simulink model "freeEvolution"  (R2023b)
settings: Solver=VariableStepAuto  StartTime=0.0  StopTime=tf  RelTol=1e-6
values from neighbouring files (symbols this model uses):
  x0 = [deg2rad(10);0]    [ShipFinStabilizers.m]    (also in plotRoutine.m)
undefined symbols (not defined in the file or in its folder): A, B, C, D, F
settings Model: Creator=valen  LastModifiedBy=valen

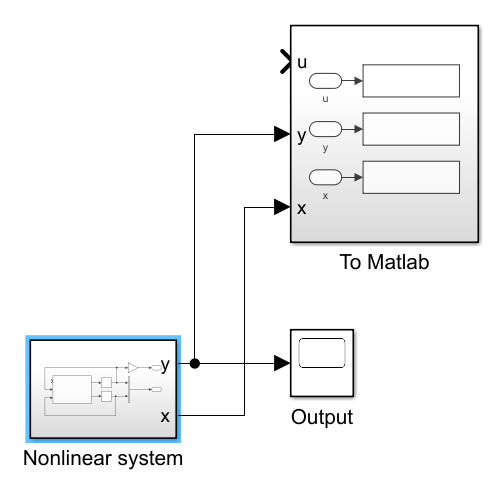
[thumbnail: Simulink's stored preview of the top-level diagram]
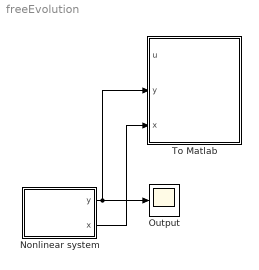
== system freeEvolution ==
  Nonlinear system : Subsystem
  Output : Scope
  To Matlab : Subsystem
  wires:
  Nonlinear system/2(x) -> To Matlab/3(x)
  Nonlinear system/1(y) -> To Matlab/2(y), Output/1

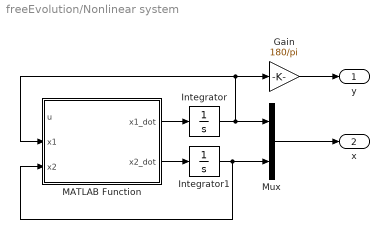
== system freeEvolution/Nonlinear system ==
  Gain : Gain  Gain=180/pi
  Integrator : Integrator  InitialCondition=x0(1)
  Integrator1 : Integrator  InitialCondition=x0(2)
  MATLAB Function : MATLAB Function  TreatAsAtomicUnit=on
  Mux : Mux  Inputs=2
  y : Outport
  x : Outport  Port=2
  wires:
  Integrator1/1 -> Mux/2, MATLAB Function/3(x2)
  Integrator/1 -> Mux/1, Gain/1, MATLAB Function/2(x1)
  MATLAB Function/2(x2_dot) -> Integrator1/1
  MATLAB Function/1(x1_dot) -> Integrator/1
  Mux/1 -> x/1
  Gain/1 -> y/1

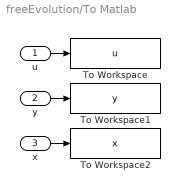
== system freeEvolution/To Matlab ==
  u : Inport  PortDimensions=1
  y : Inport  Port=2  PortDimensions=1
  x : Inport  Port=3  PortDimensions=[2,1]
  To Workspace : ToWorkspace  VariableName=u  SaveFormat=Structure With Time  SampleTime=-1
  To Workspace1 : ToWorkspace  VariableName=y  SaveFormat=Structure With Time  SampleTime=-1
  To Workspace2 : ToWorkspace  VariableName=x  SaveFormat=Structure With Time  SampleTime=-1
  wires:
  y/1 -> To Workspace1/1
  x/1 -> To Workspace2/1
  u/1 -> To Workspace/1

== matlab function freeEvolution/Nonlinear system/MATLAB Function ==
  data: u input; x1_dot output; x1 input; x2 input; x2_dot output; A parameter; B parameter; C parameter; D parameter; E parameter; F parameter
function [x1_dot,x2_dot] = ship(u,x1,x2, A, B, C, D, E, F)

    x1_dot = x2;
    x2_dot = 1/A*( B*x2 + C*x2*abs(x2) + D*x1 + E*sin(x1) + F*u);
